simulink model "openManipulatorWaypointTracking"  (R2020a)
settings: Solver=VariableStepAuto  StartTime=0.0  StopTime=12  FixedStep=0.01  RelTol=1e-3
PreLoadFcn:
  | openManipulatorParameters;
undefined symbols (not defined in the file): gripper_force, robot, waypoint_threshold, wayPoints, X, Y, Z
libraries: sm_lib x94, nesl_utility x50, OpenManipulatorLib x25, fl_lib x12, Multibody_Multiphysics_Lib x6
(part 1 of 3)
settings Model: Creator=josea  LastModifiedBy=sabir
settings DataIOCC: ReturnWorkspaceOutputs=off
settings DebuggingCC: ArithmeticOperatorsInVariantConditions=warning
settings SFSimCC: SimUseLocalCustomCode=off  CustomCodeUndefinedFunction=UseInterfaceOnly
settings RTWCC: RTWUseLocalCustomCode=off
settings SimscapeCC: SimscapeLogType=all  SimscapeLogName=simlog_waypoint_tracking  SimscapeLogLimitData=off
settings ExplorerConfigSet: InternalSimMechanicsExplorerSettings="<ExplorerConfiguration><canonicalview>default</canonicalview><AnimationSetting><BasePlaybackSpeed>1.0</BasePlaybackSpeed><PlaybackSpeedFactor>1.0</PlaybackSpeedFactor></AnimationSetting><TilePanel><TileInfo><Tiles Columns=\"1\" Count=\"1\" Rows=\"1\"><Column Weight=\"1\"/><Row Weight=\"1\"/><Tile Height=\"1\" Width=\"1\" X=\"0\" Y=\"0\"/></Tiles></TileInfo><SceneInfo><SceneViewer><BGColor><R>0.800000011920928955</R><G>0.800000011920928955</G><B>0.800000011920928955</B></BGColor><Camera><DoPerspective>on</DoPerspective><Position><X>0.660777076666317131</X><Y>0.373719867162341401</Y><Z>0.352367462185005476</Z></Position><Center><X>0.264664188667685596</X><Y>0.118807036445623571</Y><Z>0.172847607588098612</Z></Center><Up><X>-0.305288386991940719</X><Y>-0.183639326882727466</Y><Z>0.934385144568297354</Z></Up><ViewLimDist>1</ViewLimDist><YLim>0.466307658154998583</YLim><XLim>0.88035669944779904</XLim></Camera></SceneViewer></SceneInfo></TilePanel><MechEditorPanel><Cameras><Camera><Id>Camera1</Id><Value><Name>ActionCam</Name><NativeCamera><PositionKeyframeSet><Keyframe><Time>0</Time><Value><X>0.62373166555500204</X><Y>-0.42453354685624828</Y><Z>0.43384112263703245</Z></Value></Keyframe><Keyframe><Time>14</Time><Value><X>0.66077707666631713</X><Y>0.3737198671623414</Y><Z>0.35236746218500548</Z></Value></Keyframe></PositionKeyframeSet><CenterKeyframeSet><Keyframe><Time>0</Time><Value><X>0.049067643051905252</X><Y>0.14153762447470702</Y><Z>-2.0482782298048008e-06</Z></Value></Keyframe><Keyframe><Time>14</Time><Value><X>0.2646641886676856</X><Y>0.11880703644562357</Y><Z>0.17284760758809861</Z></Value></Keyframe></CenterKeyframeSet><UpVectorKeyframeSet><Keyframe><Time>0</Time><Value><X>-0.36778726768300463</X><Y>0.3009639906968779</Y><Z>0.87985976270885313</Z></Value></Keyframe><Keyframe><Time>14</Time><Value><X>-0.30528838699194072</X><Y>-0.18363932688272747</Y><Z>0.93438514456829735</Z></Value></Keyframe></UpVectorKeyframeSet></NativeCamera></Value></Camera></Cameras><GfxPanelCameraMap><MapElement CameraMLId=\"Camera1\" GfxPanelIndex=\"0\"/></GfxPanelCameraMap><VideoCreator><PlaybackSpeedRatio>1.0</PlaybackSpeedRatio><FrameRate>60</FrameRate><VideoFormat>Motion JPEG AVI</VideoFormat><FrameSize>[1366 768]</FrameSize></VideoCreator></MechEditorPanel></ExplorerConfiguration>"

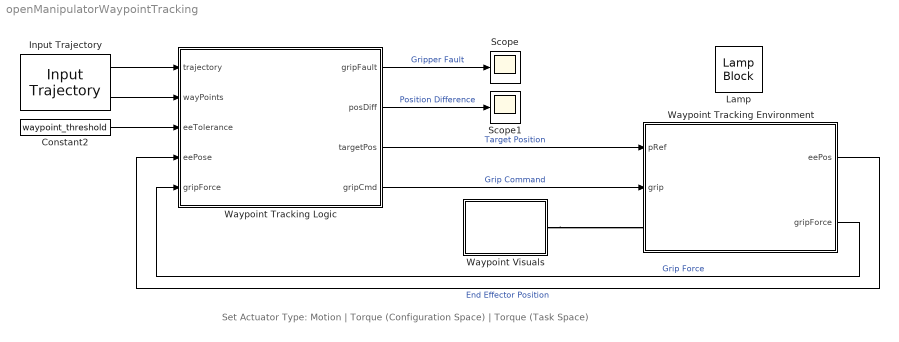
== system openManipulatorWaypointTracking ==
  note: Set Actuator Type: Motion | Torque (Configuration Space) | Torque (Task Space)
  Constant2 : Constant  Value=waypoint_threshold
  Input Trajectory : OpenManipulatorLib/Input Trajectory  numPts=50  scenarioSelection=Simple  trajSelection=Cubic
  Lamp : LampBlock
  Scope : Scope
  Scope1 : Scope
  "Waypoint Tracking Environment " : Subsystem  AncestorBlock=OpenManipulatorLib/Waypoint Tracking Environment  Variant=on  VariantControl=Variant1
      mask Display:
      | image('EnvironmentWaypointsIcon.PNG')
      | actuatorType = evalin('base','actuatorType');
      | if actuatorType == 1
      |    disp('\nMOTION')
      | elseif actuatorType == 2
      |    disp('\nTORQUE (CFG)')
      | else
      |    disp('\nTORQUE (TASK)')
      | end
  Waypoint Tracking Logic : Stateflow chart  TreatAsAtomicUnit=on
      settings: PortSchema="{\"entries\":[{\"content\":{\"sides\":[{\"content\":{\"connectorIds\":[\"In1\",\"In2\",\"In3\",\"In5\",\"In4\"]},\"type\":\"ConnectorPlacement.EquallySpacedRectSide\",\"uuid\":\"f9f3adc1-c5a5-44c6-a1d4-220b349cf5f8\"},{\"content\":{\"connectorIds\":[\"Out1\",\"Out2\",\"Out4\",\"Out3\"],\"side\":\"RIGHT\"},\"type\":\"ConnectorPlacement.EquallySpacedRectSide\",\"uuid\":\"7464d6b4-2eff-4913-ac59-da49b8f27c6f\"},{\"content\":{\"connectorIds\":[],\"side\":\"TOP\"},\"type\":\"ConnectorPlacement.EquallySpacedRectSide\",\"uuid\":\"75bc7a86-7f26-44d5-9f9e-3a119a2c8771\"}]},\"type\":\"ConnectorPlacement.EquallySpacedConnector\",\"uuid\":\"c1c5a5c7-07eb-43c1-941a-aa9e6764dbfb\"}],\"packageUris\":[\"http://schema.mathworks.com/mf0/Connector/19700101\"],\"version\":\"1.0\"}"
  Waypoint Visuals : Subsystem  mask(Waypoint and Trajectory Visualization){spherePoints=wayPoints, sphereRadius=0.01, sphereColor=[0 0.5 1], splinePoints=eePositions', splineColor=[1 0 1]}
      mask prompts: spherePoints "Sphere Positions"; sphereRadius "Sphere Radius"; sphereColor "Sphere Color"; splinePoints "Trajectory Points"; splineColor "Trajectory Color"
      mask help:
      | This dynamic subsystem places spheres on the desired waypoints and visualizes a pre-computed trajectory as a 3D spline
      |
      | Sphere Positions and Trajectory Points are both vectors for which the first 3 columns correspond to the (X, Y, Z) coordinates of the waypoints or trajectory points.
      |
      | NOTE: Make sure the library link for the subsystem is broken when copied from the library. Otherwise the mask initialization will not be able to modify the subsystem contents.
      mask init:
      | % This initialization routine deletes everything within the mask except the
      | % inport and then rebuilds the subsystem with updated information from the
      | % mask parameters
      | 
      | subsystem = gcb;
      | blocks = find_system(subsystem,'LookUnderMasks','all');
      | 
      | % Delete all previous blocks except the inport
      | for idx = 2:length(blocks)-1
      |     delete_block(blocks{idx})
      | end
      | 
      | % Delete all signals
      | while ~isempty(find_system(subsystem,'LookUnderMasks','all','FindAll','on','type','line'))
      |     lines = find_system(subsystem,'LookUnderMasks','all','FindAll','on','type','line');
      |     delete_line(lines(1))
      | end
      | 
      | %%
      | pos1 = [140 100 180 140];
      | pos2 = [140 170 180 210];
      | 
      | set_param(strcat(subsystem,'/W'),'position',[140 60 180 80])
      | 
      | % Add spline to visualize trajectory
      | add_block('sm_lib/Curves and Surfaces/Spline',strcat(subsystem,'/Trajectory Spline'));
      | set_param(strcat(subsystem,'/Trajectory Spline'),'position',pos1,'Orientation','left');
      | set_param(strcat(subsystem,'/Trajectory Spline'),'DataPoints','splinePoints','EndCOnditionType','Natural','GraphicDiffuseColor','splineColor');
      | add_line(subsystem,strcat('W','/RConn1'),strcat('Trajectory Spline','/Lconn1'));
      | 
      | % Add waypoint sphere visuals
      | for idx = 1:size(spherePoints,1)
      |     pos1 = pos1 + [60 0 60 0];
      |     pos2 = pos2 + [60 0 60 0];
      |     
      |     % Add coordinate transform and set parameters
      |     add_block('sm_lib/Frames and Transforms/Rigid Transform',strcat(subsystem,'/Rigid Transform',num2str(idx)));
      |     set_param(strcat(subsystem,'/Rigid Transform',num2str(idx)),'position',pos1,'Orientation','down');
      |     set_param(strcat(subsystem,'/Rigid Transform',num2str(idx)),'TranslationMethod','Cartesian','TranslationCartesianOffset',strcat('[',num2str(spherePoints(idx,1:3)),']'));
      |     add_line(subsystem,strcat('W','/RConn1'),strcat('Rigid Transform',num2str(idx),'/Lconn1'));
      |     
      |     % Add sphere and set parameters
      |     add_block('sm_lib/Body Elements/Spherical Solid',strcat(subsystem,'/Sphere',num2str(idx)))
      |     set_param(strcat(subsystem,'/Sphere',num2str(idx)),'position',pos2,'GraphicDiffuseColor','sphereColor','SphereRadius','sphereRadius')
      |     add_line(subsystem,strcat('Rigid Transform',num2str(idx),'/Rconn1'),strcat('Sphere',num2str(idx),'/RConn1'));
      |    
      | end
      settings: CopyFcn=set_param(gcb,'LinkStatus','breakWithoutHierarchy');
      mask DialogControl ParameterGroupVar Prompt: Sphere Parameters
      mask DialogControl Container3 Prompt: Spline Parameters
      mask Display: image('wayPointsIcon.png')
  wires:
  Input Trajectory/1 -> Waypoint Tracking Logic/1(trajectory)
  Constant2/1 -> Waypoint Tracking Logic/3(eeTolerance)
  Input Trajectory/2 -> Waypoint Tracking Logic/2(wayPoints)
  Waypoint Tracking Logic/4(targetPos) -> "Waypoint Tracking Environment "/1("pRef ")  "Target Position"
  Waypoint Tracking Logic/3(gripCmd) -> "Waypoint Tracking Environment "/2(grip)  "Grip Command"
  Waypoint Tracking Logic/2(posDiff) -> Scope1/1  "Position Difference"
  "Waypoint Tracking Environment "/1(eePos) -> Waypoint Tracking Logic/5(eePose)  "End Effector Position"
  "Waypoint Tracking Environment "/2(" gripForce") -> Waypoint Tracking Logic/4(gripForce)  "Grip Force"
  Waypoint Tracking Logic/1(gripFault) -> Scope/1  "Gripper Fault"
  connections:
  Waypoint Visuals/LConn1 -- "Waypoint Tracking Environment "/LConn1

== system openManipulatorWaypointTracking/Waypoint Tracking Environment  ==
  "pRef " : Inport
  grip : Inport  Port=2
  Motion Actuated : Subsystem  VariantControl=actuatorType==1
      mask Display: image('EnvironmentWaypointsIcon.PNG')
  Torque Actuated (Configuration Space Controller) : Subsystem  VariantControl=actuatorType==2
      mask Display: image('EnvironmentWaypointsIcon.PNG')
  Torque Actuated (Task Space Controller) : Subsystem  VariantControl=actuatorType==3
      mask Display: image('EnvironmentWaypointsIcon.PNG')
  W : PMIOPort  Side=Left
  eePos : Outport  VectorParamsAs1DForOutWhenUnconnected=off
  " gripForce" : Outport  Port=2  VectorParamsAs1DForOutWhenUnconnected=off

== system openManipulatorWaypointTracking/Waypoint Tracking Logic/saturateEE ==
  note: Saturates end effector pose based on motion limits
  desiredEE : Inport  OutDataTypeStr=double  PortDimensions=3
  f : TriggerPort  TriggerType=function-call  VariantControl=(inherit)
      settings: CopyFcn=Stateflow.SLINSF.SimulinkMan.removeBlockPreDeleteFcn  PreDeleteFcn=Stateflow.SLINSF.SimulinkMan.unsafePredeleteFcn
  Range Saturation : Subsystem  mask(End Effector Range Saturation){xUpper=0.3, xLower=0, yUpper=0.3, yLower=-0.3, zUpper=0.28, zLower=0.02}
      mask prompts: xUpper "Max X position"; xLower "Min X position"; yUpper "Max Y position"; yLower "Min Y position"; zUpper "Max Z position"; zLower "Min Z position"
      mask help: This subsystem saturates the end effector position to those within the allowable ranges for the manipulator. This prevents the inverse kinematics algorithms from attempting to find inexistent solution that timeout.
  Signal Conversion : SignalConversion  OverrideOpt=off
  maxEE : Outport  VectorParamsAs1DForOutWhenUnconnected=off
  wires:
  desiredEE/1 -> Range Saturation/1(Desired EE Pose)
  Range Saturation/1(Max EE Pose) -> Signal Conversion/1
  Signal Conversion/1 -> maxEE/1

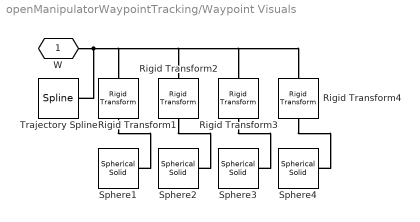
== system openManipulatorWaypointTracking/Waypoint Visuals ==
  Rigid Transform1 : sm_lib/Frames and Transforms/Rigid Transform  TranslationMethod=Cartesian  TranslationStandardOffset=0  TranslationLengthUnit=m  TranslationStandardAxis=+Z  TranslationCartesianOffset="[0.2        -0.2        0.15]"  TranslationROffset=0  TranslationROffsetUnits=m  TranslationZOffset=0  TranslationZOffsetUnits=m  TranslationThetaOffset=0  TranslationThetaOffsetUnits=deg  RotationMethod=None  RotationAngleUnits=deg  RotationStandardAxis=+Z  RotationAngle=0.0  RotationArbitraryAxis=[0 0 1]  FollAlignAxisA=+X  BaseAlignAxisA=+Y  FollAlignAxisB=+Y  BaseAlignAxisB=+Z  RotationSequenceAxes=FollowerAxes  RotationSequence=XYX  RotationSequenceAngles=[0 0 0]  RotationSequenceAnglesUnits=deg  RotationMatrix=[1 0 0; 0 1 0; 0 0 1]
  Rigid Transform2 : sm_lib/Frames and Transforms/Rigid Transform  TranslationMethod=Cartesian  TranslationStandardOffset=0  TranslationLengthUnit=m  TranslationStandardAxis=+Z  TranslationCartesianOffset="[0.2        -0.2        0.02]"  TranslationROffset=0  TranslationROffsetUnits=m  TranslationZOffset=0  TranslationZOffsetUnits=m  TranslationThetaOffset=0  TranslationThetaOffsetUnits=deg  RotationMethod=None  RotationAngleUnits=deg  RotationStandardAxis=+Z  RotationAngle=0.0  RotationArbitraryAxis=[0 0 1]  FollAlignAxisA=+X  BaseAlignAxisA=+Y  FollAlignAxisB=+Y  BaseAlignAxisB=+Z  RotationSequenceAxes=FollowerAxes  RotationSequence=XYX  RotationSequenceAngles=[0 0 0]  RotationSequenceAnglesUnits=deg  RotationMatrix=[1 0 0; 0 1 0; 0 0 1]
  Rigid Transform3 : sm_lib/Frames and Transforms/Rigid Transform  TranslationMethod=Cartesian  TranslationStandardOffset=0  TranslationLengthUnit=m  TranslationStandardAxis=+Z  TranslationCartesianOffset="[0.25           0        0.15]"  TranslationROffset=0  TranslationROffsetUnits=m  TranslationZOffset=0  TranslationZOffsetUnits=m  TranslationThetaOffset=0  TranslationThetaOffsetUnits=deg  RotationMethod=None  RotationAngleUnits=deg  RotationStandardAxis=+Z  RotationAngle=0.0  RotationArbitraryAxis=[0 0 1]  FollAlignAxisA=+X  BaseAlignAxisA=+Y  FollAlignAxisB=+Y  BaseAlignAxisB=+Z  RotationSequenceAxes=FollowerAxes  RotationSequence=XYX  RotationSequenceAngles=[0 0 0]  RotationSequenceAnglesUnits=deg  RotationMatrix=[1 0 0; 0 1 0; 0 0 1]
  Rigid Transform4 : sm_lib/Frames and Transforms/Rigid Transform  TranslationMethod=Cartesian  TranslationStandardOffset=0  TranslationLengthUnit=m  TranslationStandardAxis=+Z  TranslationCartesianOffset="[0.2         0.2        0.02]"  TranslationROffset=0  TranslationROffsetUnits=m  TranslationZOffset=0  TranslationZOffsetUnits=m  TranslationThetaOffset=0  TranslationThetaOffsetUnits=deg  RotationMethod=None  RotationAngleUnits=deg  RotationStandardAxis=+Z  RotationAngle=0.0  RotationArbitraryAxis=[0 0 1]  FollAlignAxisA=+X  BaseAlignAxisA=+Y  FollAlignAxisB=+Y  BaseAlignAxisB=+Z  RotationSequenceAxes=FollowerAxes  RotationSequence=XYX  RotationSequenceAngles=[0 0 0]  RotationSequenceAnglesUnits=deg  RotationMatrix=[1 0 0; 0 1 0; 0 0 1]
  Sphere{1..4} (4 alike) : sm_lib/Body Elements/Spherical Solid  GraphicAmbientColor=[0.15 0.15 0.15 1.0]  BasedOnType=Density  CenterOfMass=[0 0 0]  CenterOfMassUnits=m  GraphicDiffuseColor=sphereColor  Density=1000  DensityUnits=kg/m^3  DoExposeReferenceFrame=on  GraphicEmissiveColor=[0.0 0.0 0.0 1.0]  ExportEntireGeometry=off  SerializedExposedGeometries=<ExposedGeometries/>  SerializedFrames=<Frames/>  MarkerShape=Sphere  MarkerSize=10  GraphicType=FromGeometry  InertiaType=CalculateFromGeometry  Mass=1  MassUnits=kg  MomentsOfInertia=[1 1 1]  MomentsOfInertiaUnits=kg*m^2  GraphicOpacity=1.0  ProductsOfInertia=[0 0 0]  ProductsOfInertiaUnits=kg*m^2  GraphicShininess=75  GraphicSpecularColor=[0.5 0.5 0.5 1.0]  SphereRadius=sphereRadius  SphereRadiusUnits=m  GraphicVisPropType=SimpleVisualProperties
  Trajectory Spline : sm_lib/Curves and Surfaces/Spline  GraphicAmbientColor=[0.15 0.15 0.15 1.0]  GraphicDiffuseColor=splineColor  DataPoints=splinePoints  DataPointsUnits=m  GraphicEmissiveColor=[0.0 0.0 0.0 1.0]  EndConditionType=Natural  MarkerShape=Sphere  MarkerSize=10  GraphicType=FromGeometry  GraphicOpacity=1.0  GraphicShininess=75  GraphicSpecularColor=[0.5 0.5 0.5 1.0]  GraphicVisPropType=SimpleVisualProperties
  W : PMIOPort  Side=Left
  connections:
  Trajectory Spline/LConn1 -- W/RConn1 -- Rigid Transform1/LConn1 -- Rigid Transform2/LConn1 -- Rigid Transform3/LConn1 -- Rigid Transform4/LConn1
  Rigid Transform1/RConn1 -- Sphere1/RConn1
  Rigid Transform2/RConn1 -- Sphere2/RConn1
  Rigid Transform3/RConn1 -- Sphere3/RConn1
  Rigid Transform4/RConn1 -- Sphere4/RConn1

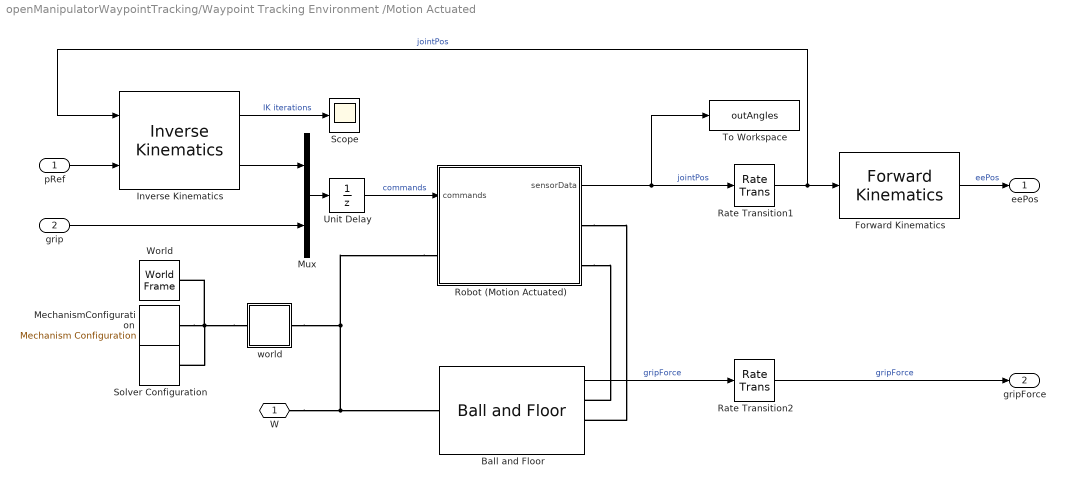
== system openManipulatorWaypointTracking/Waypoint Tracking Environment /Motion Actuated ==
  "pRef " : Inport
  grip : Inport  Port=2
  Ball and Floor : OpenManipulatorLib/Ball and Floor  PxPositionTargetValue=initPosX  PyPositionTargetValue=initPosY  PxVelocityTargetValue=initVelX  PyVelocityTargetValue=initVelY  PzPositionTargetValue=initPosZ  PzVelocityTargetValue=initVelZ
      link override Ball: GraphicDiffuseColor=[1.0 1.0 1.0]
      link override Floor: GraphicDiffuseColor=[0.6 0.8 1.0]
      link override Line: GraphicDiffuseColor=[0.6 0.6 1.0]
  Forward Kinematics : OpenManipulatorLib/Forward Kinematics  SystemSampleTime=-1  Latency=0  AutoFrameSizeCalculation=off
  Inverse Kinematics : OpenManipulatorLib/Inverse Kinematics  SystemSampleTime=-1  Latency=0  AutoFrameSizeCalculation=off
  MechanismConfiguration : sm_lib/Utilities/Mechanism Configuration  UniformGravity=Constant  GravityVector=[0 0 -9.80665]  GravityUnits=m/s^2  LinearizationDelta=0.001
  Mux : Mux  Inputs=2
  Rate Transition1 : RateTransition
  Rate Transition2 : RateTransition
  Robot (Motion Actuated) : Subsystem  AncestorBlock=|
      | OpenManipulatorLib/Robot 
      | (Motion Actuated)
      mask Display: image('RobotIcon.png')
  Scope : Scope
  Solver Configuration : nesl_utility/Solver Configuration  PhysicalDomain=network_engine_domain  SubClassName=solver  LeftPortType=input  RightPortType=generic  Tones=[]  Harmonics=[]  SimulateNoise=off  Profile=off  UseLocalSampling=off  EnableSwitchedLinearOptims=on  FrequencyDomain=off  UseCCode=off  RelTol=0.001  AbsTol=1e-06  MinStep=1e-09  ToWorkspace=off  RevertToSquareIcSolve=off  NumHomotopyIterations=100  PhasorMode=off  PhasorModeNumHarmonics=1  DoDC=off  ResidualTolerance=1e-09  UseLocalSolver=off  LocalSolverChoice=NE_BACKWARD_EULER_ADVANCER  LocalSolverSampleTime=0.001  DoFixedCost=off  MaxNonlinIter=3  MaxModeIter=2  LinearAlgebra=Sparse  EquationFormulation=NE_TIME_EF  DelaysMemoryBudget=1024  AutomaticFiltering=on  FilteringTimeConstant=0.001  PartitionStorageMethod=AS_NEEDED  PartitionMemoryBudget=1024  PartitionMethod=FAST
  To Workspace : ToWorkspace  VariableName=outAngles  SaveFormat=Structure With Time  SampleTime=0.05
  Unit Delay : UnitDelay  SampleTime=-1  HasFrameUpgradeWarning=on
  World : sm_lib/Frames and Transforms/World Frame
  world : Subsystem
  W : PMIOPort  Side=Left
  eePos : Outport  VectorParamsAs1DForOutWhenUnconnected=off
  gripForce : Outport  Port=2  VectorParamsAs1DForOutWhenUnconnected=off
  wires:
  Inverse Kinematics/2 -> Mux/1
  "pRef "/1 -> Inverse Kinematics/2
  Mux/1 -> Unit Delay/1
  grip/1 -> Mux/2
  Forward Kinematics/1 -> eePos/1  "eePos"
  Unit Delay/1 -> Robot (Motion Actuated)/1(commands)  "commands"
  Rate Transition2/1 -> gripForce/1  "gripForce"
  Rate Transition1/1 -> Forward Kinematics/1, Inverse Kinematics/1  "jointPos"
  Ball and Floor/1 -> Rate Transition2/1  "gripForce"
  Robot (Motion Actuated)/1(sensorData) -> To Workspace/1, Rate Transition1/1  "jointPos"
  Inverse Kinematics/1 -> Scope/1  "IK iterations"
  connections:
  Robot (Motion Actuated)/RConn1 -- Ball and Floor/RConn2
  Robot (Motion Actuated)/RConn2 -- Ball and Floor/RConn1
  Robot (Motion Actuated)/LConn1 -- Ball and Floor/LConn1 -- W/RConn1 -- world/RConn1
  world/LConn1 -- Solver Configuration/RConn1 -- MechanismConfiguration/RConn1 -- World/RConn1

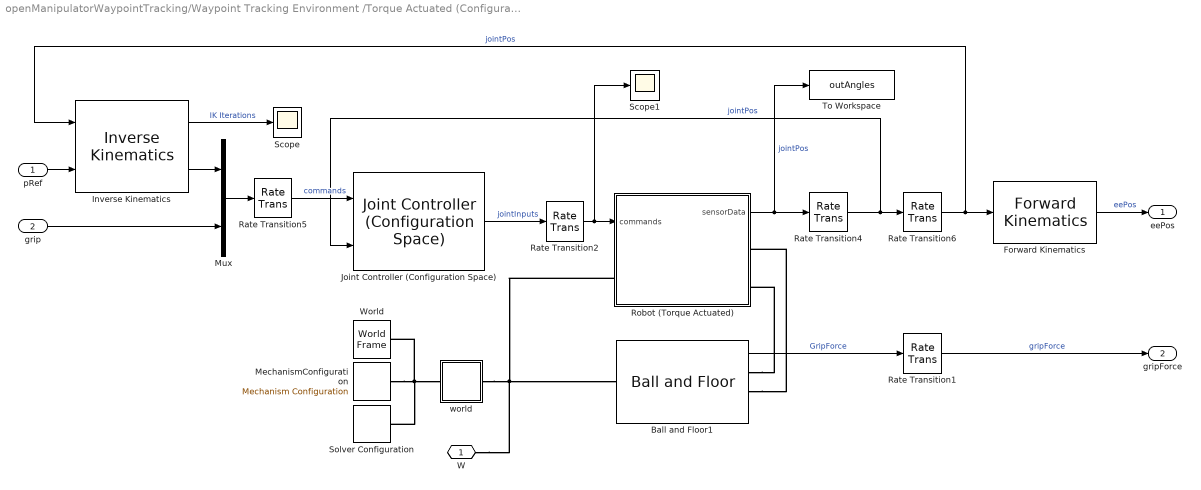
== system openManipulatorWaypointTracking/Waypoint Tracking Environment /Torque Actuated (Configuration Space Controller) ==
  "pRef " : Inport
  grip : Inport  Port=2
  Ball and Floor1 : OpenManipulatorLib/Ball and Floor  PxPositionTargetValue=initPosX  PyPositionTargetValue=initPosY  PxVelocityTargetValue=initVelX  PyVelocityTargetValue=initVelY  PzPositionTargetValue=initPosZ  PzVelocityTargetValue=initVelZ
      link override Ball: GraphicDiffuseColor=[1.0 1.0 1.0]
      link override Floor: GraphicDiffuseColor=[0.6 0.8 1.0]
      link override Line: GraphicDiffuseColor=[0.6 0.6 1.0]
  Forward Kinematics : OpenManipulatorLib/Forward Kinematics  SystemSampleTime=-1  Latency=0  AutoFrameSizeCalculation=off
  Inverse Kinematics : OpenManipulatorLib/Inverse Kinematics  SystemSampleTime=-1  Latency=0  AutoFrameSizeCalculation=off
  Joint Controller (Configuration Space) : OpenManipulatorLib/Joint Controller (Configuration Space)  SystemSampleTime=-1  VariantControl=ctrlType==1  Latency=0  AutoFrameSizeCalculation=off
  MechanismConfiguration : sm_lib/Utilities/Mechanism Configuration  UniformGravity=Constant  GravityVector=[0 0 -9.80665]  GravityUnits=m/s^2  LinearizationDelta=0.001
  Mux : Mux  Inputs=2
  Rate Transition1 : RateTransition
  Rate Transition2 : RateTransition  OutPortSampleTimeOpt=Inherit
  Rate Transition4 : RateTransition
  Rate Transition5 : RateTransition  OutPortSampleTimeOpt=Inherit
  Rate Transition6 : RateTransition
  Robot (Torque Actuated) : Subsystem  AncestorBlock=|
      | OpenManipulatorLib/Robot 
      | (Torque Actuated)
      mask Display: image('RobotIcon.png')
  Scope : Scope
  Scope1 : Scope
  Solver Configuration : nesl_utility/Solver Configuration  PhysicalDomain=network_engine_domain  SubClassName=solver  LeftPortType=input  RightPortType=generic  Tones=[]  Harmonics=[]  SimulateNoise=off  Profile=off  UseLocalSampling=off  EnableSwitchedLinearOptims=on  FrequencyDomain=off  UseCCode=off  RelTol=0.001  AbsTol=1e-06  MinStep=1e-09  ToWorkspace=off  RevertToSquareIcSolve=off  NumHomotopyIterations=100  PhasorMode=off  PhasorModeNumHarmonics=1  DoDC=off  ResidualTolerance=1e-09  UseLocalSolver=off  LocalSolverChoice=NE_BACKWARD_EULER_ADVANCER  LocalSolverSampleTime=0.001  DoFixedCost=off  MaxNonlinIter=3  MaxModeIter=2  LinearAlgebra=Sparse  EquationFormulation=NE_TIME_EF  DelaysMemoryBudget=1024  AutomaticFiltering=on  FilteringTimeConstant=0.001  PartitionStorageMethod=AS_NEEDED  PartitionMemoryBudget=1024  PartitionMethod=FAST
  To Workspace : ToWorkspace  VariableName=outAngles  SaveFormat=Structure With Time  SampleTime=0.05
  World : sm_lib/Frames and Transforms/World Frame
  world : Subsystem
  W : PMIOPort  Side=Left
  eePos : Outport  VectorParamsAs1DForOutWhenUnconnected=off
  gripForce : Outport  Port=2  VectorParamsAs1DForOutWhenUnconnected=off
  wires:
  Rate Transition5/1 -> Joint Controller (Configuration Space)/1  "commands"
  grip/1 -> Mux/2
  Inverse Kinematics/1 -> Scope/1  "IK Iterations"
  Inverse Kinematics/2 -> Mux/1
  Ball and Floor1/1 -> Rate Transition1/1  "GripForce"
  Rate Transition1/1 -> gripForce/1  "gripForce"
  Rate Transition2/1 -> Scope1/1, Robot (Torque Actuated)/1(commands)
  Joint Controller (Configuration Space)/1 -> Rate Transition2/1  "jointInputs"
  "pRef "/1 -> Inverse Kinematics/2
  Forward Kinematics/1 -> eePos/1  "eePos"
  Robot (Torque Actuated)/1(sensorData) -> To Workspace/1, Rate Transition4/1  "jointPos"
  Rate Transition4/1 -> Rate Transition6/1, Joint Controller (Configuration Space)/2  "jointPos"
  Mux/1 -> Rate Transition5/1
  Rate Transition6/1 -> Forward Kinematics/1, Inverse Kinematics/1  "jointPos"
  connections:
  World/RConn1 -- MechanismConfiguration/RConn1 -- Solver Configuration/RConn1 -- world/LConn1
  Robot (Torque Actuated)/LConn1 -- Ball and Floor1/LConn1 -- world/RConn1 -- W/RConn1
  Ball and Floor1/RConn1 -- Robot (Torque Actuated)/RConn2
  Ball and Floor1/RConn2 -- Robot (Torque Actuated)/RConn1

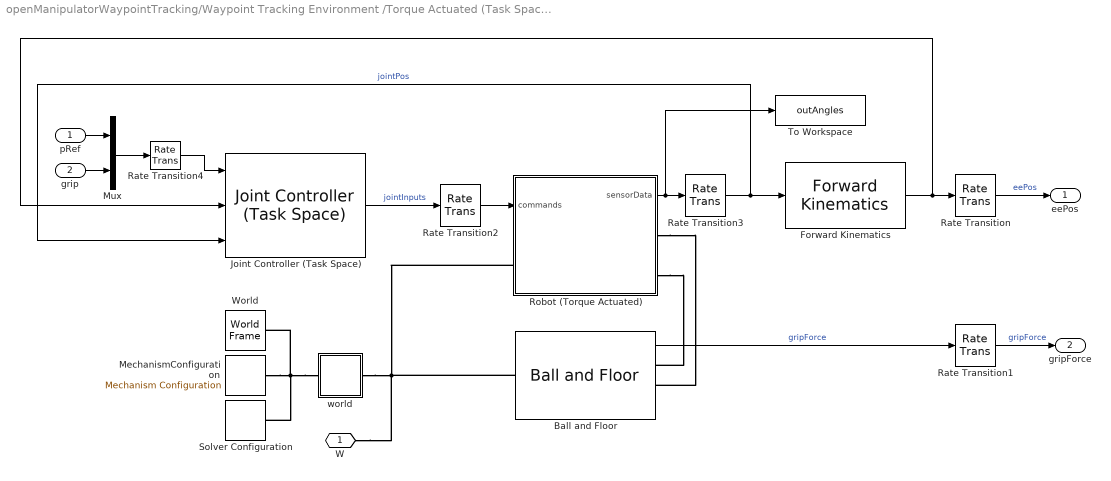
== system openManipulatorWaypointTracking/Waypoint Tracking Environment /Torque Actuated (Task Space Controller) ==
  "pRef " : Inport
  grip : Inport  Port=2
  Ball and Floor : OpenManipulatorLib/Ball and Floor  PxPositionTargetValue=initPosX  PyPositionTargetValue=initPosY  PxVelocityTargetValue=initVelX  PyVelocityTargetValue=initVelY  PzPositionTargetValue=initPosZ  PzVelocityTargetValue=initVelZ
      link override Ball: GraphicDiffuseColor=[1.0 1.0 1.0]
      link override Floor: GraphicDiffuseColor=[0.6 0.8 1.0]
      link override Line: GraphicDiffuseColor=[0.6 0.6 1.0]
  Forward Kinematics : OpenManipulatorLib/Forward Kinematics  SystemSampleTime=-1  Latency=0  AutoFrameSizeCalculation=off
  Joint Controller (Task Space) : OpenManipulatorLib/Joint Controller (Task Space)  SystemSampleTime=-1  VariantControl=ctrlType==1  Latency=0  AutoFrameSizeCalculation=off
  MechanismConfiguration : sm_lib/Utilities/Mechanism Configuration  UniformGravity=Constant  GravityVector=[0 0 -9.80665]  GravityUnits=m/s^2  LinearizationDelta=0.001
  Mux : Mux  Inputs=2
  Rate Transition{,1,3..4} (4 alike) : RateTransition
  Rate Transition2 : RateTransition  OutPortSampleTimeOpt=Inherit
  Robot (Torque Actuated) : Subsystem  AncestorBlock=|
      | OpenManipulatorLib/Robot 
      | (Torque Actuated)
      mask Display: image('RobotIcon.png')
  Solver Configuration : nesl_utility/Solver Configuration  PhysicalDomain=network_engine_domain  SubClassName=solver  LeftPortType=input  RightPortType=generic  Tones=[]  Harmonics=[]  SimulateNoise=off  Profile=off  UseLocalSampling=off  EnableSwitchedLinearOptims=on  FrequencyDomain=off  UseCCode=off  RelTol=0.001  AbsTol=1e-06  MinStep=1e-09  ToWorkspace=off  RevertToSquareIcSolve=off  NumHomotopyIterations=100  PhasorMode=off  PhasorModeNumHarmonics=1  DoDC=off  ResidualTolerance=1e-09  UseLocalSolver=off  LocalSolverChoice=NE_BACKWARD_EULER_ADVANCER  LocalSolverSampleTime=0.001  DoFixedCost=off  MaxNonlinIter=3  MaxModeIter=2  LinearAlgebra=Sparse  EquationFormulation=NE_TIME_EF  DelaysMemoryBudget=1024  AutomaticFiltering=on  FilteringTimeConstant=0.001  PartitionStorageMethod=AS_NEEDED  PartitionMemoryBudget=1024  PartitionMethod=FAST
  To Workspace : ToWorkspace  VariableName=outAngles  SaveFormat=Structure With Time  SampleTime=0.05
  World : sm_lib/Frames and Transforms/World Frame
  world : Subsystem
  W : PMIOPort  Side=Left
  eePos : Outport  VectorParamsAs1DForOutWhenUnconnected=off
  gripForce : Outport  Port=2  VectorParamsAs1DForOutWhenUnconnected=off
  wires:
  grip/1 -> Mux/2
  Mux/1 -> Rate Transition4/1
  Rate Transition3/1 -> Forward Kinematics/1, Joint Controller (Task Space)/3  "jointPos"
  Rate Transition/1 -> eePos/1  "eePos"
  Forward Kinematics/1 -> Rate Transition/1, Joint Controller (Task Space)/2
  Rate Transition4/1 -> Joint Controller (Task Space)/1
  "pRef "/1 -> Mux/1
  Joint Controller (Task Space)/1 -> Rate Transition2/1  "jointInputs"
  Rate Transition2/1 -> Robot (Torque Actuated)/1(commands)
  Rate Transition1/1 -> gripForce/1  "gripForce"
  Ball and Floor/1 -> Rate Transition1/1  "gripForce"
  Robot (Torque Actuated)/1(sensorData) -> To Workspace/1, Rate Transition3/1
  connections:
  Robot (Torque Actuated)/RConn1 -- Ball and Floor/RConn2
  Robot (Torque Actuated)/RConn2 -- Ball and Floor/RConn1
  W/RConn1 -- Robot (Torque Actuated)/LConn1 -- Ball and Floor/LConn1 -- world/RConn1
  world/LConn1 -- Solver Configuration/RConn1 -- MechanismConfiguration/RConn1 -- World/RConn1

== system openManipulatorWaypointTracking/Waypoint Tracking Logic/saturateEE/Range Saturation ==
  Desired EE Pose : Inport
  Demux : Demux  Outputs=3
  Mux : Mux  Inputs=3
  X Range : Saturate  UpperLimit=xUpper  LowerLimit=xLower
  Y Range : Saturate  UpperLimit=yUpper  LowerLimit=yLower
  Z Range : Saturate  UpperLimit=zUpper  LowerLimit=zLower
  Max EE Pose : Outport  VectorParamsAs1DForOutWhenUnconnected=off
  wires:
  Desired EE Pose/1 -> Demux/1
  Demux/2 -> Y Range/1
  Demux/3 -> Z Range/1
  X Range/1 -> Mux/1
  Mux/1 -> Max EE Pose/1
  Z Range/1 -> Mux/3
  Y Range/1 -> Mux/2
  Demux/1 -> X Range/1

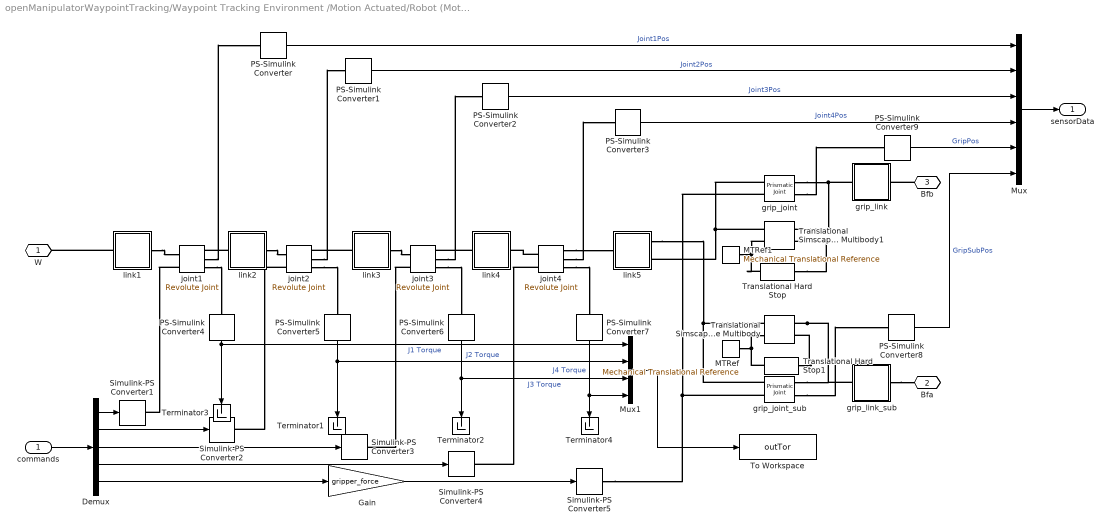
== system openManipulatorWaypointTracking/Waypoint Tracking Environment /Motion Actuated/Robot (Motion Actuated) ==
  commands : Inport
  Demux : Demux  Outputs=5
  Gain : Gain  Gain=gripper_force
  MTRef : fl_lib/Mechanical/Translational Elements/Mechanical Translational Reference
  MTRef1 : fl_lib/Mechanical/Translational Elements/Mechanical Translational Reference
  Mux : Mux  Inputs=6
  Mux1 : Mux
  PS-Simulink Converter{,1..9} (10 alike) : nesl_utility/PS-Simulink Converter  PhysicalDomain=network_engine_domain  SubClassName=ps_output  LeftPortType=input  RightPortType=output  PseudoPeriodic=off  Frequencies=[]  Unit=1  AffineConversion=off
  Simulink-PS Converter{1..5} (5 alike) : nesl_utility/Simulink-PS Converter  PhysicalDomain=network_engine_domain  SubClassName=ps_input  LeftPortType=input  RightPortType=output  PseudoPeriodic=off  Frequencies=[]  NoiseDistribution=none  NoiseParameters=[]  Unit=1  AffineConversion=off  FilteringAndDerivatives=filter  SimscapeFilterOrder=2  InputFilterTimeConstant=filter_constant  UdotUserProvided=0
  Terminator{1..4} (4 alike) : Terminator
  To Workspace : ToWorkspace  VariableName=outTor  SaveFormat=Structure With Time  SampleTime=-1
  Translational Simscape Multibody : Multibody_Multiphysics_Lib/Interfaces/Translational Simscape Multibody  SystemSampleTime=-1  Latency=0  AutoFrameSizeCalculation=off
      settings: SourceProductName=Simscape Multibody Multiphysics Library
  Translational Simscape Multibody1 : Multibody_Multiphysics_Lib/Interfaces/Translational Simscape Multibody  SystemSampleTime=-1  Latency=0  AutoFrameSizeCalculation=off
      settings: SourceProductName=Simscape Multibody Multiphysics Library
  Translational Hard Stop : fl_lib/Mechanical/Translational Elements/Translational Hard Stop  upper_bnd=0.0125 m  lower_bnd=-0.01 m  stiff_up=1e4 N/m  stiff_low=1e4 N/m  D_up=150 N/(m/s)  D_low=150 N/(m/s)  model=1  transition=0.1 mm  v_specify=off  v_priority=None  v=0 m/s  v_nominal_specify=off  v_nominal_unit=m/s  v_nominal_value=1  f_specify=off  f_priority=None  f=0 N  f_nominal_specify=off  f_nominal_unit=N  f_nominal_value=1  x_specify=off  x_priority=High  x=0 m  x_nominal_specify=off  x_nominal_unit=m  x_nominal_value=1
  Translational Hard Stop1 : fl_lib/Mechanical/Translational Elements/Translational Hard Stop  upper_bnd=0.0125 m  lower_bnd=-0.01 m  stiff_up=1e4 N/m  stiff_low=1e4 N/m  D_up=150 N/(m/s)  D_low=150 N/(m/s)  model=1  transition=0.1 mm  v_specify=off  v_priority=None  v=0 m/s  v_nominal_specify=off  v_nominal_unit=m/s  v_nominal_value=1  f_specify=off  f_priority=None  f=0 N  f_nominal_specify=off  f_nominal_unit=N  f_nominal_value=1  x_specify=off  x_priority=High  x=0 m  x_nominal_specify=off  x_nominal_unit=m  x_nominal_value=1
  grip_joint : sm_lib/Joints/Prismatic Joint  JointMode=Normal  SenseConstraintForce=off  SenseConstraintForceX=off  SenseConstraintForceY=off  SenseConstraintForceZ=off  SenseConstraintTorque=off  SenseConstraintTorqueX=off  SenseConstraintTorqueY=off  SenseConstraintTorqueZ=off  SenseTotalForce=off  SenseTotalForceX=off  SenseTotalForceY=off  SenseTotalForceZ=off  SenseTotalTorque=off  SenseTotalTorqueX=off  SenseTotalTorqueY=off  SenseTotalTorqueZ=off  CompositeWrenchDir=FollowerOnBase  CompositeWrenchFrame=BaseFrame  EquilibriumPosition=0  EquilibriumPositionUnits=m  SpringStiffness=grip_stiffness  SpringStiffnessUnits=N/m  DampingCoefficient=grip_damping  DampingCoefficientUnits=kg/s  TorqueActuationMode=InputTorque  MotionActuationMode=ComputedMotion  SensePosition=on  SenseVelocity=off  SenseAcceleration=off  SenseTorqueForce=off  SenseLowerLimitTorqueForce=off  SenseUpperLimitTorqueForce=off  LowerLimitSpecify=off  LowerLimitBound=-1  LowerLimitBoundUnits=m  LowerLimitStiffness=1e6  LowerLimitStiffnessUnits=N/m  LowerLimitDamping=1e3  LowerLimitDampingUnits=N/(m/s)  LowerLimitTransitionRegionWidth=1e-4  LowerLimitTransitionRegionWidthUnits=m  UpperLimitSpecify=off  UpperLimitBound=1  UpperLimitBoundUnits=m  UpperLimitStiffness=1e6  UpperLimitStiffnessUnits=N/m  UpperLimitDamping=1e3  UpperLimitDampingUnits=N/(m/s)  UpperLimitTransitionRegionWidth=1e-4  UpperLimitTransitionRegionWidthUnits=m  PositionTargetSpecify=off  PositionTargetPriority=High  PositionTargetValue=0  PositionTargetValueUnits=m  VelocityTargetSpecify=off  VelocityTargetPriority=High  VelocityTargetValue=0  VelocityTargetValueUnits=m/s
  grip_joint_sub : sm_lib/Joints/Prismatic Joint  JointMode=Normal  SenseConstraintForce=off  SenseConstraintForceX=off  SenseConstraintForceY=off  SenseConstraintForceZ=off  SenseConstraintTorque=off  SenseConstraintTorqueX=off  SenseConstraintTorqueY=off  SenseConstraintTorqueZ=off  SenseTotalForce=off  SenseTotalForceX=off  SenseTotalForceY=off  SenseTotalForceZ=off  SenseTotalTorque=off  SenseTotalTorqueX=off  SenseTotalTorqueY=off  SenseTotalTorqueZ=off  CompositeWrenchDir=FollowerOnBase  CompositeWrenchFrame=BaseFrame  EquilibriumPosition=0  EquilibriumPositionUnits=m  SpringStiffness=grip_stiffness  SpringStiffnessUnits=N/m  DampingCoefficient=grip_damping  DampingCoefficientUnits=kg/s  TorqueActuationMode=InputTorque  MotionActuationMode=ComputedMotion  SensePosition=on  SenseVelocity=off  SenseAcceleration=off  SenseTorqueForce=off  SenseLowerLimitTorqueForce=off  SenseUpperLimitTorqueForce=off  LowerLimitSpecify=off  LowerLimitBound=-1  LowerLimitBoundUnits=m  LowerLimitStiffness=1e6  LowerLimitStiffnessUnits=N/m  LowerLimitDamping=1e3  LowerLimitDampingUnits=N/(m/s)  LowerLimitTransitionRegionWidth=1e-4  LowerLimitTransitionRegionWidthUnits=m  UpperLimitSpecify=off  UpperLimitBound=1  UpperLimitBoundUnits=m  UpperLimitStiffness=1e6  UpperLimitStiffnessUnits=N/m  UpperLimitDamping=1e3  UpperLimitDampingUnits=N/(m/s)  UpperLimitTransitionRegionWidth=1e-4  UpperLimitTransitionRegionWidthUnits=m  PositionTargetSpecify=off  PositionTargetPriority=High  PositionTargetValue=0  PositionTargetValueUnits=m  VelocityTargetSpecify=off  VelocityTargetPriority=High  VelocityTargetValue=0  VelocityTargetValueUnits=m/s
  grip_link : Subsystem
  grip_link_sub : Subsystem
  joint{1..4} (4 alike) : sm_lib/Joints/Revolute Joint  JointMode=Normal  SenseConstraintForce=off  SenseConstraintForceX=off  SenseConstraintForceY=off  SenseConstraintForceZ=off  SenseConstraintTorque=off  SenseConstraintTorqueX=off  SenseConstraintTorqueY=off  SenseConstraintTorqueZ=off  SenseTotalForce=off  SenseTotalForceX=off  SenseTotalForceY=off  SenseTotalForceZ=off  SenseTotalTorque=off  SenseTotalTorqueX=off  SenseTotalTorqueY=off  SenseTotalTorqueZ=off  CompositeWrenchDir=FollowerOnBase  CompositeWrenchFrame=BaseFrame  EquilibriumPosition=0  EquilibriumPositionUnits=deg  SpringStiffness=0  SpringStiffnessUnits=N*m/deg  DampingCoefficient=joint_damping  DampingCoefficientUnits=N*m/(rad/s)  TorqueActuationMode=ComputedTorque  MotionActuationMode=InputMotion  SensePosition=on  SenseVelocity=off  SenseAcceleration=off  SenseTorqueForce=on  SenseLowerLimitTorqueForce=off  SenseUpperLimitTorqueForce=off  LowerLimitSpecify=off  LowerLimitBound=-90  LowerLimitBoundUnits=deg  LowerLimitStiffness=1e4  LowerLimitStiffnessUnits=N*m/deg  LowerLimitDamping=10  LowerLimitDampingUnits=N*m/(deg/s)  LowerLimitTransitionRegionWidth=0.1  LowerLimitTransitionRegionWidthUnits=deg  UpperLimitSpecify=off  UpperLimitBound=90  UpperLimitBoundUnits=deg  UpperLimitStiffness=1e4  UpperLimitStiffnessUnits=N*m/deg  UpperLimitDamping=10  UpperLimitDampingUnits=N*m/(deg/s)  UpperLimitTransitionRegionWidth=0.1  UpperLimitTransitionRegionWidthUnits=deg  PositionTargetSpecify=off  PositionTargetPriority=High  PositionTargetValue=0  PositionTargetValueUnits=deg  VelocityTargetSpecify=off  VelocityTargetPriority=High  VelocityTargetValue=0  VelocityTargetValueUnits=deg/s
  link1 : Subsystem
  link2 : Subsystem
  link3 : Subsystem
  link4 : Subsystem
  link5 : Subsystem
  W : PMIOPort  Side=Left
  Bfa : PMIOPort  Port=2  Side=Right
  Bfb : PMIOPort  Port=3  Side=Right
  sensorData : Outport  VectorParamsAs1DForOutWhenUnconnected=off
  wires:
  Demux/5 -> Gain/1
  PS-Simulink Converter7/1 -> Mux1/4, Terminator4/1  "J4 Torque"
  PS-Simulink Converter6/1 -> Mux1/3, Terminator2/1  "J3 Torque"
  PS-Simulink Converter5/1 -> Terminator1/1, Mux1/2  "J2 Torque"
  PS-Simulink Converter4/1 -> Mux1/1, Terminator3/1  "J1 Torque"
  commands/1 -> Demux/1
  PS-Simulink Converter/1 -> Mux/1  "Joint1Pos"
  PS-Simulink Converter1/1 -> Mux/2  "Joint2Pos"
  PS-Simulink Converter2/1 -> Mux/3  "Joint3Pos"
  PS-Simulink Converter3/1 -> Mux/4  "Joint4Pos"
  Gain/1 -> Simulink-PS Converter5/1
  Mux/1 -> sensorData/1
  Demux/4 -> Simulink-PS Converter4/1
  Demux/2 -> Simulink-PS Converter2/1
  Demux/1 -> Simulink-PS Converter1/1
  Demux/3 -> Simulink-PS Converter3/1
  PS-Simulink Converter8/1 -> Mux/6  "GripSubPos"
  PS-Simulink Converter9/1 -> Mux/5  "GripPos"
  Mux1/1 -> To Workspace/1
  connections:
  joint4/RConn3 -- PS-Simulink Converter7/LConn1
  joint3/RConn3 -- PS-Simulink Converter6/LConn1
  joint2/RConn3 -- PS-Simulink Converter5/LConn1
  joint1/RConn3 -- PS-Simulink Converter4/LConn1
  joint4/RConn1 -- link5/LConn1
  link1/RConn1 -- joint1/LConn1
  link2/RConn1 -- joint2/LConn1
  link3/RConn1 -- joint3/LConn1
  link3/LConn1 -- joint2/RConn1
  link1/LConn1 -- W/RConn1
  link2/LConn1 -- joint1/RConn1
  joint4/LConn1 -- link4/RConn1
  link4/LConn1 -- joint3/RConn1
  joint3/RConn2 -- PS-Simulink Converter2/LConn1
  joint4/RConn2 -- PS-Simulink Converter3/LConn1
  joint2/LConn2 -- Simulink-PS Converter2/RConn1
  joint4/LConn2 -- Simulink-PS Converter4/RConn1
  joint3/LConn2 -- Simulink-PS Converter3/RConn1
  joint1/LConn2 -- Simulink-PS Converter1/RConn1
  joint2/RConn2 -- PS-Simulink Converter1/LConn1
  joint1/RConn2 -- PS-Simulink Converter/LConn1
  Translational Simscape Multibody/RConn1 -- grip_link_sub/LConn1 -- grip_joint_sub/RConn1
  MTRef/LConn1 -- Translational Hard Stop1/RConn1 -- Translational Simscape Multibody/LConn2
  MTRef1/LConn1 -- Translational Hard Stop/RConn1 -- Translational Simscape Multibody1/LConn2
  grip_joint/RConn1 -- grip_link/LConn1 -- Translational Simscape Multibody1/RConn1
  grip_joint_sub/LConn1 -- link5/RConn1 -- Translational Simscape Multibody/LConn1
  grip_joint/LConn1 -- link5/RConn2 -- Translational Simscape Multibody1/LConn1
  grip_joint/RConn2 -- PS-Simulink Converter9/LConn1
  grip_joint/LConn2 -- grip_joint_sub/LConn2 -- Simulink-PS Converter5/RConn1
  grip_joint_sub/RConn2 -- PS-Simulink Converter8/LConn1
  Translational Hard Stop/LConn1 -- Translational Simscape Multibody1/RConn2
  Translational Hard Stop1/LConn1 -- Translational Simscape Multibody/RConn2
  Bfb/RConn1 -- grip_link/RConn1
  grip_link_sub/RConn1 -- Bfa/RConn1

== system openManipulatorWaypointTracking/Waypoint Tracking Environment /Motion Actuated/world ==
  ReferenceFrame : sm_lib/Frames and Transforms/Reference Frame
  world_fixed_OriginTransform : sm_lib/Frames and Transforms/Rigid Transform  TranslationMethod=Cartesian  TranslationStandardOffset=0  TranslationLengthUnit=m  TranslationStandardAxis=+Z  TranslationCartesianOffset=[0, 0, 0]  TranslationROffset=0  TranslationROffsetUnits=m  TranslationZOffset=0  TranslationZOffsetUnits=m  TranslationThetaOffset=0  TranslationThetaOffsetUnits=deg  RotationMethod=RotationSequence  RotationAngleUnits=deg  RotationStandardAxis=+Z  RotationAngle=0.0  RotationArbitraryAxis=[0 0 1]  FollAlignAxisA=+X  BaseAlignAxisA=+Y  FollAlignAxisB=+Y  BaseAlignAxisB=+Z  RotationSequenceAxes=BaseAxes  RotationSequence=XYZ  RotationSequenceAngles=[0, 0, 0]  RotationSequenceAnglesUnits=rad  RotationMatrix=[1 0 0; 0 1 0; 0 0 1]
  F : PMIOPort  Side=Left
  F1 : PMIOPort  Port=2  Side=Right
  connections:
  world_fixed_OriginTransform/RConn1 -- F1/RConn1
  F/RConn1 -- ReferenceFrame/RConn1 -- world_fixed_OriginTransform/LConn1
